simulink model "LinearPlant"  (R2020a)
settings: Solver=VariableStepAuto  StartTime=0.0  StopTime=10.0  RelTol=1e-3
settings Model: Creator=liamw  LastModifiedBy=liamw

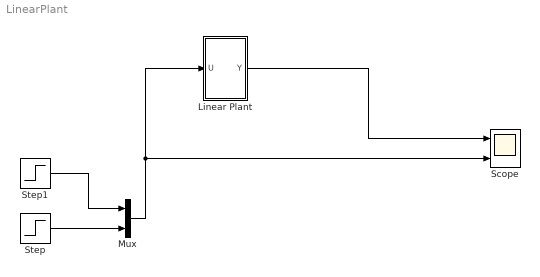
== system LinearPlant ==
  Linear Plant : Subsystem
  Mux : Mux  Inputs=2
  Scope : Scope  NumInputPorts=2
  Step : Step  SampleTime=0
  Step1 : Step  After=0  SampleTime=0
  wires:
  Mux/1 -> Scope/2, Linear Plant/1(U)
  Step/1 -> Mux/2
  Step1/1 -> Mux/1
  Linear Plant/1(Y) -> Scope/1

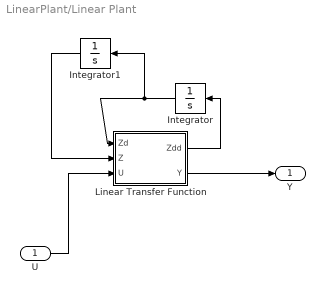
== system LinearPlant/Linear Plant ==
  U : Inport
  Integrator : Integrator
  Integrator1 : Integrator
  Linear Transfer Function : MATLAB Function  TreatAsAtomicUnit=on
  Y : Outport
  wires:
  Linear Transfer Function/2(Y) -> Y/1
  Linear Transfer Function/1(Zdd) -> Integrator/1
  U/1 -> Linear Transfer Function/3(U)
  Integrator/1 -> Integrator1/1, Linear Transfer Function/1(Zd)
  Integrator1/1 -> Linear Transfer Function/2(Z)

== matlab function LinearPlant/Linear Plant/Linear Transfer Function ==
  data: Zd input; Z input; U input; Zdd output; Y output
function [Zdd, Y]  = fcn(Zd, Z, U)
%% House keeping
Zdd=zeros(3,1);
Y = zeros(2,1);

%% System Constants
I = 0.0008;
m = 0.35;
r = 0.03;
k = 50;
ko = 200;
b = 0.09;
bo = 0.5;


%% Calculate a new alpha
a = 0.523599; % 30 degrees in radians


%% System Matrices
M = [I 0 0;
     0 I 0;
     0 0 m];
 
B = [b 0 0;
     0 b 0;
     0 0 bo];
 
Knl = [1.5*k*r^2, -1.5*k*r^2, -k*r*cos(a);
       -1.5*k*r^2, 1.5*k*r^2, k*r*cos(a);
       -k*r*cos(a), k*r*cos(a), ko+2*k*cos(a)*cos(a)];
   
% Get the right size input   
Ua = [1 0;
      0 1;
      0 0]*U;

Zdd = (M^-1)*Ua - (M^-1)*B*Zd - (M^-1)*Knl*Z;

% Get the output we want
Y = [((Zd(1,1)+Zd(2,1))/2);   % Average of motor speeds
     Z(3,1)];                 % Tension
